simulink model "adsorption1"  (R2022b)
settings: Solver=VariableStepAuto  StartTime=0.0  StopTime=3600  RelTol=1e-3
libraries: fl_lib x171, nesl_utility x44
(part 1 of 2)
settings Model: Creator=kulka  LastModifiedBy=kulka

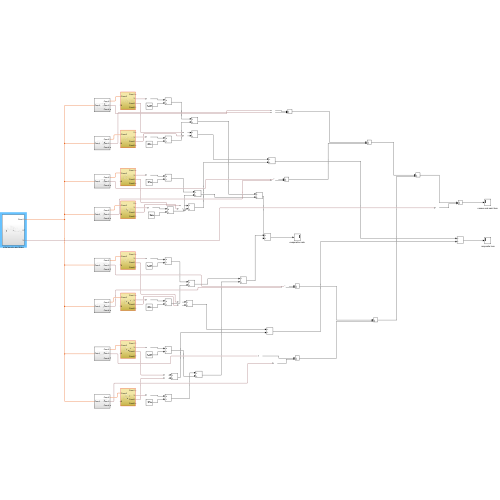
[thumbnail: Simulink's stored preview of the top-level diagram]
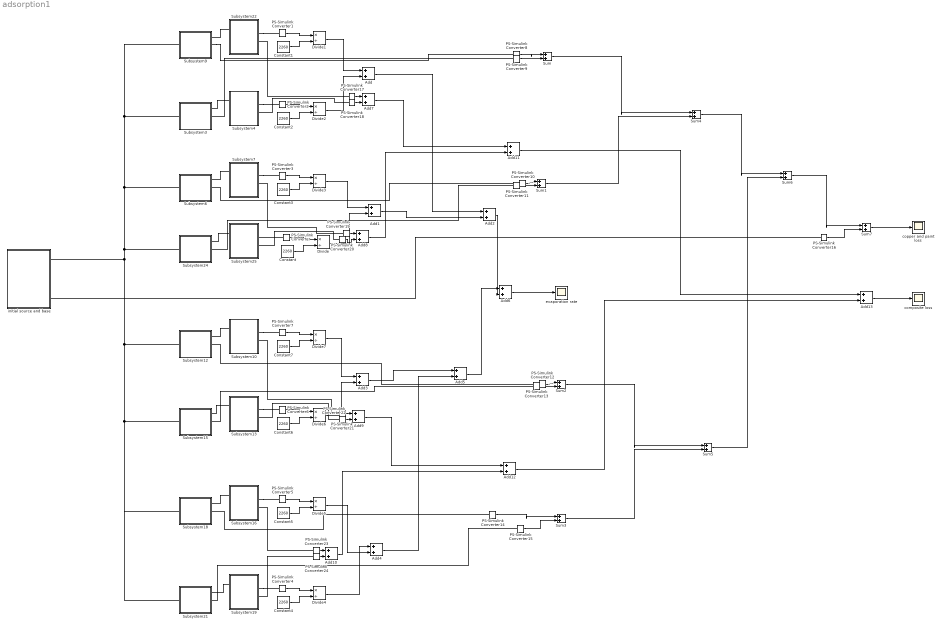
== system adsorption1 ==
  Add{,1..13} (14 alike) : Sum
  Constant{,1..7} (8 alike) : Constant  Value=2260
  Divide{,1..7} (8 alike) : Product  Inputs=*/  RndMeth=Zero  SaturateOnIntegerOverflow=on
  PS-Simulink Converter{,1..24} (25 alike) : nesl_utility/PS-Simulink Converter  PhysicalDomain=network_engine_domain  SubClassName=ps_output  LeftPortType=input  RightPortType=output  PseudoPeriodic=off  Frequencies=[]  VectorFormat=inherit  Unit=inherit  AffineConversion=off
  Subsystem10 : Subsystem
  Subsystem12 : Subsystem
  Subsystem13 : Subsystem
  Subsystem15 : Subsystem
  Subsystem16 : Subsystem
  Subsystem18 : Subsystem
  Subsystem19 : Subsystem
  Subsystem21 : Subsystem
  Subsystem22 : Subsystem
  Subsystem24 : Subsystem
  Subsystem25 : Subsystem
  Subsystem3 : Subsystem
  Subsystem4 : Subsystem
  Subsystem6 : Subsystem
  Subsystem7 : Subsystem
  Subsystem9 : Subsystem
  Sum{,1..7} (8 alike) : Sum  Inputs=|++
  composite loss : Scope
  copper and paint loss : Scope
  evaporation rate : Scope
  initial source and base : Subsystem
  wires:
  Constant/1 -> Divide/2
  PS-Simulink Converter/1 -> Divide/1
  PS-Simulink Converter1/1 -> Divide1/1
  Constant1/1 -> Divide1/2
  PS-Simulink Converter2/1 -> Divide2/1
  Constant2/1 -> Divide2/2
  PS-Simulink Converter3/1 -> Divide3/1
  Constant3/1 -> Divide3/2
  PS-Simulink Converter4/1 -> Divide4/1
  Constant4/1 -> Divide4/2
  PS-Simulink Converter5/1 -> Divide5/1
  Constant5/1 -> Divide5/2
  PS-Simulink Converter6/1 -> Divide6/1
  Constant6/1 -> Divide6/2
  PS-Simulink Converter7/1 -> Divide7/1
  Constant7/1 -> Divide7/2
  Divide1/1 -> Add/1
  Divide2/1 -> Add/2
  Divide3/1 -> Add1/1
  Divide/1 -> Add1/2
  Add/1 -> Add2/1
  Add1/1 -> Add2/2
  Divide7/1 -> Add3/1
  Divide6/1 -> Add3/2
  Divide5/1 -> Add4/2
  Divide4/1 -> Add4/1
  Add4/1 -> Add5/2
  Add3/1 -> Add5/1
  Add2/1 -> Add6/2
  Add5/1 -> Add6/1
  Add6/1 -> evaporation rate/1
  PS-Simulink Converter8/1 -> Sum/1
  PS-Simulink Converter9/1 -> Sum/2
  PS-Simulink Converter10/1 -> Sum1/1
  PS-Simulink Converter11/1 -> Sum1/2
  Sum/1 -> Sum4/1
  Sum1/1 -> Sum4/2
  Sum4/1 -> Sum6/1
  PS-Simulink Converter12/1 -> Sum2/1
  PS-Simulink Converter13/1 -> Sum2/2
  PS-Simulink Converter14/1 -> Sum3/1
  PS-Simulink Converter15/1 -> Sum3/2
  Sum3/1 -> Sum5/2
  Sum2/1 -> Sum5/1
  Sum5/1 -> Sum6/2
  Sum6/1 -> Sum7/1
  PS-Simulink Converter16/1 -> Sum7/2
  Sum7/1 -> copper and paint loss/1
  Add13/1 -> composite loss/1
  PS-Simulink Converter17/1 -> Add7/1
  PS-Simulink Converter18/1 -> Add7/2
  Add7/1 -> Add11/1
  PS-Simulink Converter19/1 -> Add8/1
  PS-Simulink Converter20/1 -> Add8/2
  Add8/1 -> Add11/2
  Add11/1 -> Add13/1
  PS-Simulink Converter21/1 -> Add9/1
  PS-Simulink Converter22/1 -> Add9/2
  Add9/1 -> Add12/1
  PS-Simulink Converter23/1 -> Add10/1
  PS-Simulink Converter24/1 -> Add10/2
  Add10/1 -> Add12/2
  Add12/1 -> Add13/2
  connections:
  Subsystem22/LConn1 -- Subsystem9/RConn1
  Subsystem4/LConn1 -- Subsystem3/RConn1
  Subsystem7/LConn1 -- Subsystem6/RConn1
  Subsystem25/LConn1 -- Subsystem24/RConn1
  Subsystem10/LConn1 -- Subsystem12/RConn1
  Subsystem13/LConn1 -- Subsystem15/RConn1
  Subsystem16/LConn1 -- Subsystem18/RConn1
  Subsystem21/LConn1 -- Subsystem18/LConn1 -- Subsystem15/LConn1 -- Subsystem12/LConn1 -- Subsystem24/LConn1 -- Subsystem6/LConn1 -- Subsystem9/LConn1 -- Subsystem3/LConn1 -- initial source and base/RConn1
  Subsystem19/LConn1 -- Subsystem21/RConn1
  PS-Simulink Converter/LConn1 -- Subsystem25/RConn2
  Subsystem22/RConn2 -- PS-Simulink Converter1/LConn1
  Subsystem4/RConn2 -- PS-Simulink Converter2/LConn1
  Subsystem7/RConn2 -- PS-Simulink Converter3/LConn1
  Subsystem19/RConn2 -- PS-Simulink Converter4/LConn1
  Subsystem16/RConn2 -- PS-Simulink Converter5/LConn1
  Subsystem13/RConn2 -- PS-Simulink Converter6/LConn1
  Subsystem10/RConn2 -- PS-Simulink Converter7/LConn1
  Subsystem9/RConn2 -- PS-Simulink Converter8/LConn1
  PS-Simulink Converter9/LConn1 -- Subsystem3/RConn2
  PS-Simulink Converter10/LConn1 -- Subsystem6/RConn2
  PS-Simulink Converter11/LConn1 -- Subsystem24/RConn2
  PS-Simulink Converter12/LConn1 -- Subsystem12/RConn2
  PS-Simulink Converter13/LConn1 -- Subsystem15/RConn2
  PS-Simulink Converter14/LConn1 -- Subsystem18/RConn2
  PS-Simulink Converter15/LConn1 -- Subsystem21/RConn2
  PS-Simulink Converter16/LConn1 -- initial source and base/RConn3
  PS-Simulink Converter17/LConn1 -- Subsystem22/RConn3
  PS-Simulink Converter18/LConn1 -- Subsystem4/RConn3
  PS-Simulink Converter19/LConn1 -- Subsystem7/RConn3
  PS-Simulink Converter20/LConn1 -- Subsystem25/RConn3
  PS-Simulink Converter21/LConn1 -- Subsystem10/RConn3
  PS-Simulink Converter22/LConn1 -- Subsystem13/RConn3
  PS-Simulink Converter23/LConn1 -- Subsystem16/RConn3
  PS-Simulink Converter24/LConn1 -- Subsystem19/RConn3

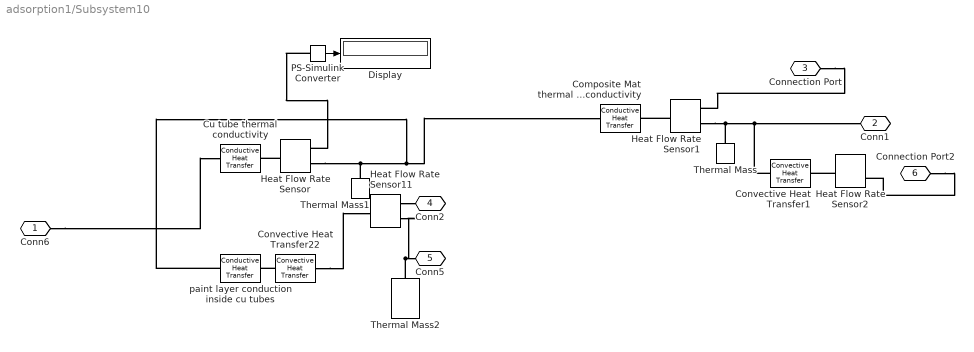
== system adsorption1/Subsystem10 ==
  Composite Mat thermal conductivity : fl_lib/Thermal/Thermal Elements/Conductive Heat Transfer  thermal_type=foundation.enum.ConstantVariableTabulated.Constant  wall_geometry=foundation.enum.ConductionWallGeometry.Planar  area=4186.1715e-6 m^2  thickness=0.002 m  d_in=0.05 m  d_out=0.1 m  L=1 m  th_cond_min=10 W/(K*m)  th_cond=0.1 W/(K*m)  th_cond_TLU=[413, 401, 392, 383, 371, 357, 342] W/(K*m)  temp_TLU=[200, 273, 400, 600, 800, 1000, 1200] K  T_specify=off  T_priority=None  T=0 K  T_nominal_specify=off  T_nominal_unit=K  T_nominal_value=1  Q_specify=on  Q_priority=None  Q=0 W  Q_nominal_specify=on  Q_nominal_unit=W  Q_nominal_value=1
  Convective Heat Transfer1 : fl_lib/Thermal/Thermal Elements/Convective Heat Transfer  thermal_type=foundation.enum.constant_variable.constant  area=4186.1715e-6 m^2  heat_tr_coeff=8 W/(K*m^2)  min_heat_tr_coeff=1e-3 W/(K*m^2)  T_specify=off  T_priority=None  T=0 K  T_nominal_specify=off  T_nominal_unit=K  T_nominal_value=1  Q_specify=on  Q_priority=None  Q=0 W  Q_nominal_specify=on  Q_nominal_unit=W  Q_nominal_value=1
  Convective Heat Transfer22 : fl_lib/Thermal/Thermal Elements/Convective Heat Transfer  thermal_type=foundation.enum.constant_variable.constant  area=3086.6125e-6 m^2  heat_tr_coeff=20 W/(K*m^2)  min_heat_tr_coeff=1e-3 W/(K*m^2)  T_specify=off  T_priority=None  T=0 K  T_nominal_specify=off  T_nominal_unit=K  T_nominal_value=1  Q_specify=on  Q_priority=None  Q=0 W  Q_nominal_specify=on  Q_nominal_unit=W  Q_nominal_value=1
  Cu tube thermal conductivity : fl_lib/Thermal/Thermal Elements/Conductive Heat Transfer  thermal_type=foundation.enum.ConstantVariableTabulated.Constant  wall_geometry=foundation.enum.ConductionWallGeometry.Planar  area=1.3744e-4 m^2  thickness=0.07 m  d_in=0.05 m  d_out=0.1 m  L=1 m  th_cond_min=10 W/(K*m)  th_cond=398 W/(K*m)  th_cond_TLU=[413, 401, 392, 383, 371, 357, 342] W/(K*m)  temp_TLU=[200, 273, 400, 600, 800, 1000, 1200] K  T_specify=off  T_priority=None  T=0 K  T_nominal_specify=off  T_nominal_unit=K  T_nominal_value=1  Q_specify=on  Q_priority=None  Q=0 W  Q_nominal_specify=on  Q_nominal_unit=W  Q_nominal_value=1
  Display : Display
  Heat Flow Rate Sensor{,1..2,11} (4 alike) : fl_lib/Thermal/Thermal Sensors/Heat Flow Rate Sensor
  PS-Simulink Converter : nesl_utility/PS-Simulink Converter  PhysicalDomain=network_engine_domain  SubClassName=ps_output  LeftPortType=input  RightPortType=output  PseudoPeriodic=off  Frequencies=[]  VectorFormat=inherit  Unit=inherit  AffineConversion=off
  Thermal Mass : fl_lib/Thermal/Thermal Elements/Thermal Mass  mass=6.6727e-2 kg  sp_heat=150 J/(K*kg)  num_ports=foundation.enum.numPorts2.one  T_specify=off  T_priority=High  T=300 K  T_nominal_specify=off  T_nominal_unit=K  T_nominal_value=1  Q_specify=off  Q_priority=None  Q=0 W  Q_nominal_specify=off  Q_nominal_unit=W  Q_nominal_value=1
  Thermal Mass1 : fl_lib/Thermal/Thermal Elements/Thermal Mass  mass=3.7865e-2 kg  sp_heat=390 J/(K*kg)  num_ports=foundation.enum.numPorts2.one  T_specify=off  T_priority=High  T=300 K  T_nominal_specify=off  T_nominal_unit=K  T_nominal_value=1  Q_specify=off  Q_priority=None  Q=0 W  Q_nominal_specify=off  Q_nominal_unit=W  Q_nominal_value=1
  Thermal Mass2 : fl_lib/Thermal/Thermal Elements/Thermal Mass  mass=0.001 kg  sp_heat=1000 J/(K*kg)  num_ports=foundation.enum.numPorts2.one  T_specify=off  T_priority=High  T=300 K  T_nominal_specify=off  T_nominal_unit=K  T_nominal_value=1  Q_specify=off  Q_priority=None  Q=0 W  Q_nominal_specify=off  Q_nominal_unit=W  Q_nominal_value=1
  paint layer conduction inside cu tubes : fl_lib/Thermal/Thermal Elements/Conductive Heat Transfer  thermal_type=foundation.enum.ConstantVariableTabulated.Constant  wall_geometry=foundation.enum.ConductionWallGeometry.Planar  area=3086.6125e-5 m^2  thickness=0.001 m  d_in=0.05 m  d_out=0.1 m  L=1 m  th_cond_min=10 W/(K*m)  th_cond=0.1 W/(K*m)  th_cond_TLU=[413, 401, 392, 383, 371, 357, 342] W/(K*m)  temp_TLU=[200, 273, 400, 600, 800, 1000, 1200] K  T_specify=off  T_priority=None  T=0 K  T_nominal_specify=off  T_nominal_unit=K  T_nominal_value=1  Q_specify=on  Q_priority=None  Q=0 W  Q_nominal_specify=on  Q_nominal_unit=W  Q_nominal_value=1
  Conn6 : PMIOPort  Side=Left
  Conn1 : PMIOPort  Port=2  Side=Right
  Connection Port : PMIOPort  Port=3  Side=Right
  Conn2 : PMIOPort  Port=4  Side=Right
  Conn5 : PMIOPort  Port=5  Side=Right
  Connection Port2 : PMIOPort  Port=6  Side=Left
  wires:
  PS-Simulink Converter/1 -> Display/1
  connections:
  Heat Flow Rate Sensor11/RConn1 -- Conn2/RConn1
  Conn6/RConn1 -- Cu tube thermal conductivity/LConn1
  Heat Flow Rate Sensor11/RConn2 -- Thermal Mass2/LConn1 -- Conn5/RConn1
  Convective Heat Transfer22/RConn1 -- Heat Flow Rate Sensor11/LConn1
  Convective Heat Transfer22/LConn1 -- paint layer conduction inside cu tubes/RConn1
  Heat Flow Rate Sensor/LConn1 -- Cu tube thermal conductivity/RConn1
  PS-Simulink Converter/LConn1 -- Heat Flow Rate Sensor/RConn1
  Heat Flow Rate Sensor/RConn2 -- Thermal Mass1/LConn1 -- paint layer conduction inside cu tubes/LConn1 -- Composite Mat thermal conductivity/LConn1
  Heat Flow Rate Sensor1/LConn1 -- Composite Mat thermal conductivity/RConn1
  Heat Flow Rate Sensor1/RConn2 -- Thermal Mass/LConn1 -- Convective Heat Transfer1/LConn1 -- Conn1/RConn1
  Connection Port/RConn1 -- Heat Flow Rate Sensor1/RConn1
  Connection Port2/RConn1 -- Heat Flow Rate Sensor2/RConn2
  Heat Flow Rate Sensor2/LConn1 -- Convective Heat Transfer1/RConn1

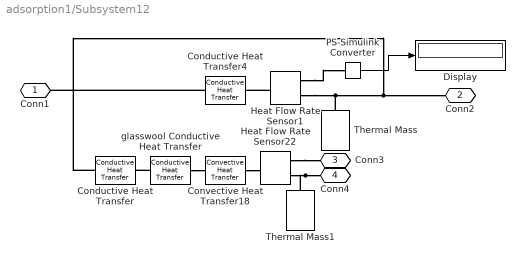
== system adsorption1/Subsystem12 ==
  Conductive Heat Transfer : fl_lib/Thermal/Thermal Elements/Conductive Heat Transfer  thermal_type=foundation.enum.ConstantVariableTabulated.Constant  wall_geometry=foundation.enum.ConductionWallGeometry.Planar  area=1.14e-3 m^2  thickness=0.02 m  d_in=0.05 m  d_out=0.1 m  L=1 m  th_cond_min=10 W/(K*m)  th_cond=0.1 W/(K*m)  th_cond_TLU=[413, 401, 392, 383, 371, 357, 342] W/(K*m)  temp_TLU=[200, 273, 400, 600, 800, 1000, 1200] K  T_specify=off  T_priority=None  T=0 K  T_nominal_specify=off  T_nominal_unit=K  T_nominal_value=1  Q_specify=on  Q_priority=None  Q=0 W  Q_nominal_specify=on  Q_nominal_unit=W  Q_nominal_value=1
  Conductive Heat Transfer4 : fl_lib/Thermal/Thermal Elements/Conductive Heat Transfer  thermal_type=foundation.enum.ConstantVariableTabulated.Constant  wall_geometry=foundation.enum.ConductionWallGeometry.Planar  area=1.14e-3 m^2  thickness=0.02 m  d_in=0.05 m  d_out=0.1 m  L=1 m  th_cond_min=10 W/(K*m)  th_cond=398 W/(K*m)  th_cond_TLU=[413, 401, 392, 383, 371, 357, 342] W/(K*m)  temp_TLU=[200, 273, 400, 600, 800, 1000, 1200] K  T_specify=off  T_priority=None  T=0 K  T_nominal_specify=off  T_nominal_unit=K  T_nominal_value=1  Q_specify=on  Q_priority=None  Q=0 W  Q_nominal_specify=on  Q_nominal_unit=W  Q_nominal_value=1
  Convective Heat Transfer18 : fl_lib/Thermal/Thermal Elements/Convective Heat Transfer  thermal_type=foundation.enum.constant_variable.constant  area=1.14e-3 m^2  heat_tr_coeff=12 W/(K*m^2)  min_heat_tr_coeff=1e-3 W/(K*m^2)  T_specify=off  T_priority=None  T=0 K  T_nominal_specify=off  T_nominal_unit=K  T_nominal_value=1  Q_specify=on  Q_priority=None  Q=0 W  Q_nominal_specify=on  Q_nominal_unit=W  Q_nominal_value=1
  Display : Display
  Heat Flow Rate Sensor1 : fl_lib/Thermal/Thermal Sensors/Heat Flow Rate Sensor
  Heat Flow Rate Sensor22 : fl_lib/Thermal/Thermal Sensors/Heat Flow Rate Sensor
  PS-Simulink Converter : nesl_utility/PS-Simulink Converter  PhysicalDomain=network_engine_domain  SubClassName=ps_output  LeftPortType=input  RightPortType=output  PseudoPeriodic=off  Frequencies=[]  VectorFormat=inherit  Unit=inherit  AffineConversion=off
  Thermal Mass : fl_lib/Thermal/Thermal Elements/Thermal Mass  mass=(0.20178)-(1.885e-6) kg  sp_heat=390 J/(K*kg)  num_ports=foundation.enum.numPorts2.one  T_specify=off  T_priority=High  T=300 K  T_nominal_specify=off  T_nominal_unit=K  T_nominal_value=1  Q_specify=off  Q_priority=None  Q=0 W  Q_nominal_specify=off  Q_nominal_unit=W  Q_nominal_value=1
  Thermal Mass1 : fl_lib/Thermal/Thermal Elements/Thermal Mass  mass=0.001 kg  sp_heat=1000 J/(K*kg)  num_ports=foundation.enum.numPorts2.one  T_specify=off  T_priority=High  T=300 K  T_nominal_specify=off  T_nominal_unit=K  T_nominal_value=1  Q_specify=off  Q_priority=None  Q=0 W  Q_nominal_specify=off  Q_nominal_unit=W  Q_nominal_value=1
  glasswool Conductive Heat Transfer : fl_lib/Thermal/Thermal Elements/Conductive Heat Transfer  thermal_type=foundation.enum.ConstantVariableTabulated.Constant  wall_geometry=foundation.enum.ConductionWallGeometry.Planar  area=3e-3 m^2  thickness=5e-3 m  d_in=0.05 m  d_out=0.1 m  L=1 m  th_cond_min=10 W/(K*m)  th_cond=0.032 W/(K*m)  th_cond_TLU=[413, 401, 392, 383, 371, 357, 342] W/(K*m)  temp_TLU=[200, 273, 400, 600, 800, 1000, 1200] K  T_specify=off  T_priority=None  T=0 K  T_nominal_specify=off  T_nominal_unit=K  T_nominal_value=1  Q_specify=on  Q_priority=None  Q=0 W  Q_nominal_specify=on  Q_nominal_unit=W  Q_nominal_value=1
  Conn1 : PMIOPort  Side=Left
  Conn2 : PMIOPort  Port=2  Side=Right
  Conn3 : PMIOPort  Port=3  Side=Right
  Conn4 : PMIOPort  Port=4  Side=Right
  wires:
  PS-Simulink Converter/1 -> Display/1
  connections:
  Conductive Heat Transfer4/LConn1 -- Conn1/RConn1
  Convective Heat Transfer18/RConn1 -- Heat Flow Rate Sensor22/LConn1
  Heat Flow Rate Sensor22/RConn2 -- Thermal Mass1/LConn1 -- Conn4/RConn1
  Heat Flow Rate Sensor22/RConn1 -- Conn3/RConn1
  Heat Flow Rate Sensor1/LConn1 -- Conductive Heat Transfer4/RConn1
  Heat Flow Rate Sensor1/RConn2 -- Thermal Mass/LConn1 -- Conductive Heat Transfer/LConn1 -- Conn2/RConn1
  Heat Flow Rate Sensor1/RConn1 -- PS-Simulink Converter/LConn1
  glasswool Conductive Heat Transfer/LConn1 -- Conductive Heat Transfer/RConn1
  glasswool Conductive Heat Transfer/RConn1 -- Convective Heat Transfer18/LConn1

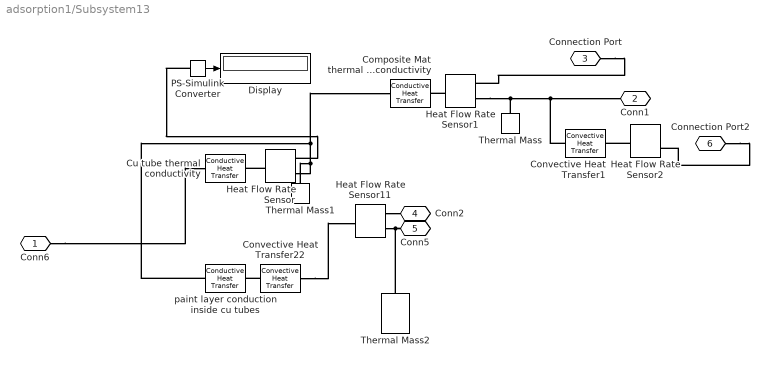
== system adsorption1/Subsystem13 ==
  Composite Mat thermal conductivity : fl_lib/Thermal/Thermal Elements/Conductive Heat Transfer  thermal_type=foundation.enum.ConstantVariableTabulated.Constant  wall_geometry=foundation.enum.ConductionWallGeometry.Planar  area=4186.1715e-6 m^2  thickness=0.002 m  d_in=0.05 m  d_out=0.1 m  L=1 m  th_cond_min=10 W/(K*m)  th_cond=0.1 W/(K*m)  th_cond_TLU=[413, 401, 392, 383, 371, 357, 342] W/(K*m)  temp_TLU=[200, 273, 400, 600, 800, 1000, 1200] K  T_specify=off  T_priority=None  T=0 K  T_nominal_specify=off  T_nominal_unit=K  T_nominal_value=1  Q_specify=on  Q_priority=None  Q=0 W  Q_nominal_specify=on  Q_nominal_unit=W  Q_nominal_value=1
  Convective Heat Transfer1 : fl_lib/Thermal/Thermal Elements/Convective Heat Transfer  thermal_type=foundation.enum.constant_variable.constant  area=4186.1715e-6 m^2  heat_tr_coeff=8 W/(K*m^2)  min_heat_tr_coeff=1e-3 W/(K*m^2)  T_specify=off  T_priority=None  T=0 K  T_nominal_specify=off  T_nominal_unit=K  T_nominal_value=1  Q_specify=on  Q_priority=None  Q=0 W  Q_nominal_specify=on  Q_nominal_unit=W  Q_nominal_value=1
  Convective Heat Transfer22 : fl_lib/Thermal/Thermal Elements/Convective Heat Transfer  thermal_type=foundation.enum.constant_variable.constant  area=3086.6125e-6 m^2  heat_tr_coeff=20 W/(K*m^2)  min_heat_tr_coeff=1e-3 W/(K*m^2)  T_specify=off  T_priority=None  T=0 K  T_nominal_specify=off  T_nominal_unit=K  T_nominal_value=1  Q_specify=on  Q_priority=None  Q=0 W  Q_nominal_specify=on  Q_nominal_unit=W  Q_nominal_value=1
  Cu tube thermal conductivity : fl_lib/Thermal/Thermal Elements/Conductive Heat Transfer  thermal_type=foundation.enum.ConstantVariableTabulated.Constant  wall_geometry=foundation.enum.ConductionWallGeometry.Planar  area=1.3744e-4 m^2  thickness=0.07 m  d_in=0.05 m  d_out=0.1 m  L=1 m  th_cond_min=10 W/(K*m)  th_cond=398 W/(K*m)  th_cond_TLU=[413, 401, 392, 383, 371, 357, 342] W/(K*m)  temp_TLU=[200, 273, 400, 600, 800, 1000, 1200] K  T_specify=off  T_priority=None  T=0 K  T_nominal_specify=off  T_nominal_unit=K  T_nominal_value=1  Q_specify=on  Q_priority=None  Q=0 W  Q_nominal_specify=on  Q_nominal_unit=W  Q_nominal_value=1
  Display : Display
  Heat Flow Rate Sensor{,1..2,11} (4 alike) : fl_lib/Thermal/Thermal Sensors/Heat Flow Rate Sensor
  PS-Simulink Converter : nesl_utility/PS-Simulink Converter  PhysicalDomain=network_engine_domain  SubClassName=ps_output  LeftPortType=input  RightPortType=output  PseudoPeriodic=off  Frequencies=[]  VectorFormat=inherit  Unit=inherit  AffineConversion=off
  Thermal Mass : fl_lib/Thermal/Thermal Elements/Thermal Mass  mass=6.6727e-2 kg  sp_heat=150 J/(K*kg)  num_ports=foundation.enum.numPorts2.one  T_specify=off  T_priority=High  T=300 K  T_nominal_specify=off  T_nominal_unit=K  T_nominal_value=1  Q_specify=off  Q_priority=None  Q=0 W  Q_nominal_specify=off  Q_nominal_unit=W  Q_nominal_value=1
  Thermal Mass1 : fl_lib/Thermal/Thermal Elements/Thermal Mass  mass=3.7865e-2 kg  sp_heat=390 J/(K*kg)  num_ports=foundation.enum.numPorts2.one  T_specify=off  T_priority=High  T=300 K  T_nominal_specify=off  T_nominal_unit=K  T_nominal_value=1  Q_specify=off  Q_priority=None  Q=0 W  Q_nominal_specify=off  Q_nominal_unit=W  Q_nominal_value=1
  Thermal Mass2 : fl_lib/Thermal/Thermal Elements/Thermal Mass  mass=0.001 kg  sp_heat=1000 J/(K*kg)  num_ports=foundation.enum.numPorts2.one  T_specify=off  T_priority=High  T=300 K  T_nominal_specify=off  T_nominal_unit=K  T_nominal_value=1  Q_specify=off  Q_priority=None  Q=0 W  Q_nominal_specify=off  Q_nominal_unit=W  Q_nominal_value=1
  paint layer conduction inside cu tubes : fl_lib/Thermal/Thermal Elements/Conductive Heat Transfer  thermal_type=foundation.enum.ConstantVariableTabulated.Constant  wall_geometry=foundation.enum.ConductionWallGeometry.Planar  area=3086.6125e-5 m^2  thickness=0.001 m  d_in=0.05 m  d_out=0.1 m  L=1 m  th_cond_min=10 W/(K*m)  th_cond=0.1 W/(K*m)  th_cond_TLU=[413, 401, 392, 383, 371, 357, 342] W/(K*m)  temp_TLU=[200, 273, 400, 600, 800, 1000, 1200] K  T_specify=off  T_priority=None  T=0 K  T_nominal_specify=off  T_nominal_unit=K  T_nominal_value=1  Q_specify=on  Q_priority=None  Q=0 W  Q_nominal_specify=on  Q_nominal_unit=W  Q_nominal_value=1
  Conn6 : PMIOPort  Side=Left
  Conn1 : PMIOPort  Port=2  Side=Right
  Connection Port : PMIOPort  Port=3  Side=Right
  Conn2 : PMIOPort  Port=4  Side=Right
  Conn5 : PMIOPort  Port=5  Side=Right
  Connection Port2 : PMIOPort  Port=6  Side=Left
  wires:
  PS-Simulink Converter/1 -> Display/1
  connections:
  Heat Flow Rate Sensor11/RConn1 -- Conn2/RConn1
  Conn6/RConn1 -- Cu tube thermal conductivity/LConn1
  Heat Flow Rate Sensor11/RConn2 -- Thermal Mass2/LConn1 -- Conn5/RConn1
  Convective Heat Transfer22/RConn1 -- Heat Flow Rate Sensor11/LConn1
  Convective Heat Transfer22/LConn1 -- paint layer conduction inside cu tubes/RConn1
  Heat Flow Rate Sensor/LConn1 -- Cu tube thermal conductivity/RConn1
  PS-Simulink Converter/LConn1 -- Heat Flow Rate Sensor/RConn1
  Heat Flow Rate Sensor/RConn2 -- Thermal Mass1/LConn1 -- paint layer conduction inside cu tubes/LConn1 -- Composite Mat thermal conductivity/LConn1
  Heat Flow Rate Sensor1/LConn1 -- Composite Mat thermal conductivity/RConn1
  Heat Flow Rate Sensor1/RConn2 -- Thermal Mass/LConn1 -- Convective Heat Transfer1/LConn1 -- Conn1/RConn1
  Connection Port/RConn1 -- Heat Flow Rate Sensor1/RConn1
  Connection Port2/RConn1 -- Heat Flow Rate Sensor2/RConn2
  Heat Flow Rate Sensor2/LConn1 -- Convective Heat Transfer1/RConn1

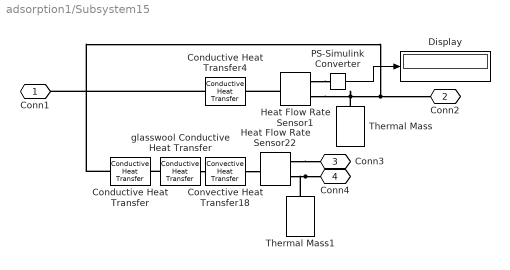
== system adsorption1/Subsystem15 ==
  Conductive Heat Transfer : fl_lib/Thermal/Thermal Elements/Conductive Heat Transfer  thermal_type=foundation.enum.ConstantVariableTabulated.Constant  wall_geometry=foundation.enum.ConductionWallGeometry.Planar  area=2*1.14e-3 m^2  thickness=0.02*2 m  d_in=0.05 m  d_out=0.1 m  L=1 m  th_cond_min=10 W/(K*m)  th_cond=0.1 W/(K*m)  th_cond_TLU=[413, 401, 392, 383, 371, 357, 342] W/(K*m)  temp_TLU=[200, 273, 400, 600, 800, 1000, 1200] K  T_specify=off  T_priority=None  T=0 K  T_nominal_specify=off  T_nominal_unit=K  T_nominal_value=1  Q_specify=on  Q_priority=None  Q=0 W  Q_nominal_specify=on  Q_nominal_unit=W  Q_nominal_value=1
  Conductive Heat Transfer4 : fl_lib/Thermal/Thermal Elements/Conductive Heat Transfer  thermal_type=foundation.enum.ConstantVariableTabulated.Constant  wall_geometry=foundation.enum.ConductionWallGeometry.Planar  area=2*1.14e-3 m^2  thickness=0.02*2 m  d_in=0.05 m  d_out=0.1 m  L=1 m  th_cond_min=10 W/(K*m)  th_cond=398 W/(K*m)  th_cond_TLU=[413, 401, 392, 383, 371, 357, 342] W/(K*m)  temp_TLU=[200, 273, 400, 600, 800, 1000, 1200] K  T_specify=off  T_priority=None  T=0 K  T_nominal_specify=off  T_nominal_unit=K  T_nominal_value=1  Q_specify=on  Q_priority=None  Q=0 W  Q_nominal_specify=on  Q_nominal_unit=W  Q_nominal_value=1
  Convective Heat Transfer18 : fl_lib/Thermal/Thermal Elements/Convective Heat Transfer  thermal_type=foundation.enum.constant_variable.constant  area=1.14e-3 m^2  heat_tr_coeff=12 W/(K*m^2)  min_heat_tr_coeff=1e-3 W/(K*m^2)  T_specify=off  T_priority=None  T=0 K  T_nominal_specify=off  T_nominal_unit=K  T_nominal_value=1  Q_specify=on  Q_priority=None  Q=0 W  Q_nominal_specify=on  Q_nominal_unit=W  Q_nominal_value=1
  Display : Display
  Heat Flow Rate Sensor1 : fl_lib/Thermal/Thermal Sensors/Heat Flow Rate Sensor
  Heat Flow Rate Sensor22 : fl_lib/Thermal/Thermal Sensors/Heat Flow Rate Sensor
  PS-Simulink Converter : nesl_utility/PS-Simulink Converter  PhysicalDomain=network_engine_domain  SubClassName=ps_output  LeftPortType=input  RightPortType=output  PseudoPeriodic=off  Frequencies=[]  VectorFormat=inherit  Unit=inherit  AffineConversion=off
  Thermal Mass : fl_lib/Thermal/Thermal Elements/Thermal Mass  mass=(2*0.20178)-(2*1.885e-6) kg  sp_heat=390 J/(K*kg)  num_ports=foundation.enum.numPorts2.one  T_specify=off  T_priority=High  T=300 K  T_nominal_specify=off  T_nominal_unit=K  T_nominal_value=1  Q_specify=off  Q_priority=None  Q=0 W  Q_nominal_specify=off  Q_nominal_unit=W  Q_nominal_value=1
  Thermal Mass1 : fl_lib/Thermal/Thermal Elements/Thermal Mass  mass=0.001 kg  sp_heat=1000 J/(K*kg)  num_ports=foundation.enum.numPorts2.one  T_specify=off  T_priority=High  T=300 K  T_nominal_specify=off  T_nominal_unit=K  T_nominal_value=1  Q_specify=off  Q_priority=None  Q=0 W  Q_nominal_specify=off  Q_nominal_unit=W  Q_nominal_value=1
  glasswool Conductive Heat Transfer : fl_lib/Thermal/Thermal Elements/Conductive Heat Transfer  thermal_type=foundation.enum.ConstantVariableTabulated.Constant  wall_geometry=foundation.enum.ConductionWallGeometry.Planar  area=3e-3 m^2  thickness=5e-3 m  d_in=0.05 m  d_out=0.1 m  L=1 m  th_cond_min=10 W/(K*m)  th_cond=0.032 W/(K*m)  th_cond_TLU=[413, 401, 392, 383, 371, 357, 342] W/(K*m)  temp_TLU=[200, 273, 400, 600, 800, 1000, 1200] K  T_specify=off  T_priority=None  T=0 K  T_nominal_specify=off  T_nominal_unit=K  T_nominal_value=1  Q_specify=on  Q_priority=None  Q=0 W  Q_nominal_specify=on  Q_nominal_unit=W  Q_nominal_value=1
  Conn1 : PMIOPort  Side=Left
  Conn2 : PMIOPort  Port=2  Side=Right
  Conn3 : PMIOPort  Port=3  Side=Right
  Conn4 : PMIOPort  Port=4  Side=Right
  wires:
  PS-Simulink Converter/1 -> Display/1
  connections:
  Conductive Heat Transfer4/LConn1 -- Conn1/RConn1
  Convective Heat Transfer18/RConn1 -- Heat Flow Rate Sensor22/LConn1
  Heat Flow Rate Sensor22/RConn2 -- Thermal Mass1/LConn1 -- Conn4/RConn1
  Heat Flow Rate Sensor22/RConn1 -- Conn3/RConn1
  Heat Flow Rate Sensor1/LConn1 -- Conductive Heat Transfer4/RConn1
  Heat Flow Rate Sensor1/RConn2 -- Thermal Mass/LConn1 -- Conductive Heat Transfer/LConn1 -- Conn2/RConn1
  Heat Flow Rate Sensor1/RConn1 -- PS-Simulink Converter/LConn1
  glasswool Conductive Heat Transfer/LConn1 -- Conductive Heat Transfer/RConn1
  glasswool Conductive Heat Transfer/RConn1 -- Convective Heat Transfer18/LConn1

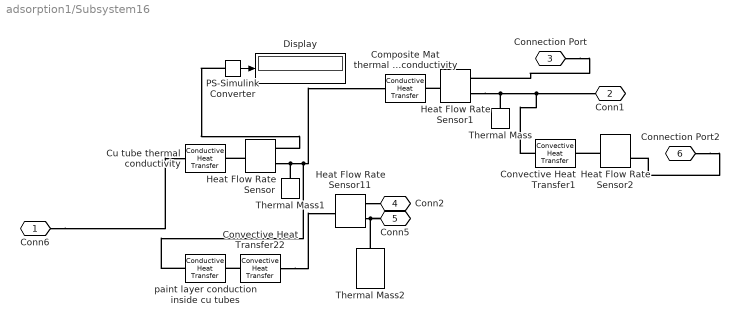
== system adsorption1/Subsystem16 ==
  Composite Mat thermal conductivity : fl_lib/Thermal/Thermal Elements/Conductive Heat Transfer  thermal_type=foundation.enum.ConstantVariableTabulated.Constant  wall_geometry=foundation.enum.ConductionWallGeometry.Planar  area=4186.1715e-6 m^2  thickness=0.002 m  d_in=0.05 m  d_out=0.1 m  L=1 m  th_cond_min=10 W/(K*m)  th_cond=0.1 W/(K*m)  th_cond_TLU=[413, 401, 392, 383, 371, 357, 342] W/(K*m)  temp_TLU=[200, 273, 400, 600, 800, 1000, 1200] K  T_specify=off  T_priority=None  T=0 K  T_nominal_specify=off  T_nominal_unit=K  T_nominal_value=1  Q_specify=on  Q_priority=None  Q=0 W  Q_nominal_specify=on  Q_nominal_unit=W  Q_nominal_value=1
  Convective Heat Transfer1 : fl_lib/Thermal/Thermal Elements/Convective Heat Transfer  thermal_type=foundation.enum.constant_variable.constant  area=4186.1715e-6 m^2  heat_tr_coeff=8 W/(K*m^2)  min_heat_tr_coeff=1e-3 W/(K*m^2)  T_specify=off  T_priority=None  T=0 K  T_nominal_specify=off  T_nominal_unit=K  T_nominal_value=1  Q_specify=on  Q_priority=None  Q=0 W  Q_nominal_specify=on  Q_nominal_unit=W  Q_nominal_value=1
  Convective Heat Transfer22 : fl_lib/Thermal/Thermal Elements/Convective Heat Transfer  thermal_type=foundation.enum.constant_variable.constant  area=3086.6125e-6 m^2  heat_tr_coeff=20 W/(K*m^2)  min_heat_tr_coeff=1e-3 W/(K*m^2)  T_specify=off  T_priority=None  T=0 K  T_nominal_specify=off  T_nominal_unit=K  T_nominal_value=1  Q_specify=on  Q_priority=None  Q=0 W  Q_nominal_specify=on  Q_nominal_unit=W  Q_nominal_value=1
  Cu tube thermal conductivity : fl_lib/Thermal/Thermal Elements/Conductive Heat Transfer  thermal_type=foundation.enum.ConstantVariableTabulated.Constant  wall_geometry=foundation.enum.ConductionWallGeometry.Planar  area=1.3744e-4 m^2  thickness=0.07 m  d_in=0.05 m  d_out=0.1 m  L=1 m  th_cond_min=10 W/(K*m)  th_cond=398 W/(K*m)  th_cond_TLU=[413, 401, 392, 383, 371, 357, 342] W/(K*m)  temp_TLU=[200, 273, 400, 600, 800, 1000, 1200] K  T_specify=off  T_priority=None  T=0 K  T_nominal_specify=off  T_nominal_unit=K  T_nominal_value=1  Q_specify=on  Q_priority=None  Q=0 W  Q_nominal_specify=on  Q_nominal_unit=W  Q_nominal_value=1
  Display : Display
  Heat Flow Rate Sensor{,1..2,11} (4 alike) : fl_lib/Thermal/Thermal Sensors/Heat Flow Rate Sensor
  PS-Simulink Converter : nesl_utility/PS-Simulink Converter  PhysicalDomain=network_engine_domain  SubClassName=ps_output  LeftPortType=input  RightPortType=output  PseudoPeriodic=off  Frequencies=[]  VectorFormat=inherit  Unit=inherit  AffineConversion=off
  Thermal Mass : fl_lib/Thermal/Thermal Elements/Thermal Mass  mass=6.6727e-2 kg  sp_heat=150 J/(K*kg)  num_ports=foundation.enum.numPorts2.one  T_specify=off  T_priority=High  T=300 K  T_nominal_specify=off  T_nominal_unit=K  T_nominal_value=1  Q_specify=off  Q_priority=None  Q=0 W  Q_nominal_specify=off  Q_nominal_unit=W  Q_nominal_value=1
  Thermal Mass1 : fl_lib/Thermal/Thermal Elements/Thermal Mass  mass=3.7865e-2 kg  sp_heat=390 J/(K*kg)  num_ports=foundation.enum.numPorts2.one  T_specify=off  T_priority=High  T=300 K  T_nominal_specify=off  T_nominal_unit=K  T_nominal_value=1  Q_specify=off  Q_priority=None  Q=0 W  Q_nominal_specify=off  Q_nominal_unit=W  Q_nominal_value=1
  Thermal Mass2 : fl_lib/Thermal/Thermal Elements/Thermal Mass  mass=0.001 kg  sp_heat=1000 J/(K*kg)  num_ports=foundation.enum.numPorts2.one  T_specify=off  T_priority=High  T=300 K  T_nominal_specify=off  T_nominal_unit=K  T_nominal_value=1  Q_specify=off  Q_priority=None  Q=0 W  Q_nominal_specify=off  Q_nominal_unit=W  Q_nominal_value=1
  paint layer conduction inside cu tubes : fl_lib/Thermal/Thermal Elements/Conductive Heat Transfer  thermal_type=foundation.enum.ConstantVariableTabulated.Constant  wall_geometry=foundation.enum.ConductionWallGeometry.Planar  area=3086.6125e-5 m^2  thickness=0.001 m  d_in=0.05 m  d_out=0.1 m  L=1 m  th_cond_min=10 W/(K*m)  th_cond=0.1 W/(K*m)  th_cond_TLU=[413, 401, 392, 383, 371, 357, 342] W/(K*m)  temp_TLU=[200, 273, 400, 600, 800, 1000, 1200] K  T_specify=off  T_priority=None  T=0 K  T_nominal_specify=off  T_nominal_unit=K  T_nominal_value=1  Q_specify=on  Q_priority=None  Q=0 W  Q_nominal_specify=on  Q_nominal_unit=W  Q_nominal_value=1
  Conn6 : PMIOPort  Side=Left
  Conn1 : PMIOPort  Port=2  Side=Right
  Connection Port : PMIOPort  Port=3  Side=Right
  Conn2 : PMIOPort  Port=4  Side=Right
  Conn5 : PMIOPort  Port=5  Side=Right
  Connection Port2 : PMIOPort  Port=6  Side=Left
  wires:
  PS-Simulink Converter/1 -> Display/1
  connections:
  Heat Flow Rate Sensor11/RConn1 -- Conn2/RConn1
  Conn6/RConn1 -- Cu tube thermal conductivity/LConn1
  Heat Flow Rate Sensor11/RConn2 -- Thermal Mass2/LConn1 -- Conn5/RConn1
  Convective Heat Transfer22/RConn1 -- Heat Flow Rate Sensor11/LConn1
  Convective Heat Transfer22/LConn1 -- paint layer conduction inside cu tubes/RConn1
  Heat Flow Rate Sensor/LConn1 -- Cu tube thermal conductivity/RConn1
  PS-Simulink Converter/LConn1 -- Heat Flow Rate Sensor/RConn1
  Heat Flow Rate Sensor/RConn2 -- Thermal Mass1/LConn1 -- paint layer conduction inside cu tubes/LConn1 -- Composite Mat thermal conductivity/LConn1
  Heat Flow Rate Sensor1/LConn1 -- Composite Mat thermal conductivity/RConn1
  Heat Flow Rate Sensor1/RConn2 -- Thermal Mass/LConn1 -- Convective Heat Transfer1/LConn1 -- Conn1/RConn1
  Connection Port/RConn1 -- Heat Flow Rate Sensor1/RConn1
  Connection Port2/RConn1 -- Heat Flow Rate Sensor2/RConn2
  Heat Flow Rate Sensor2/LConn1 -- Convective Heat Transfer1/RConn1

== system adsorption1/Subsystem18 ==
  Conductive Heat Transfer : fl_lib/Thermal/Thermal Elements/Conductive Heat Transfer  thermal_type=foundation.enum.ConstantVariableTabulated.Constant  wall_geometry=foundation.enum.ConductionWallGeometry.Planar  area=3*1.14e-3 m^2  thickness=0.02*3 m  d_in=0.05 m  d_out=0.1 m  L=1 m  th_cond_min=10 W/(K*m)  th_cond=0.1 W/(K*m)  th_cond_TLU=[413, 401, 392, 383, 371, 357, 342] W/(K*m)  temp_TLU=[200, 273, 400, 600, 800, 1000, 1200] K  T_specify=off  T_priority=None  T=0 K  T_nominal_specify=off  T_nominal_unit=K  T_nominal_value=1  Q_specify=on  Q_priority=None  Q=0 W  Q_nominal_specify=on  Q_nominal_unit=W  Q_nominal_value=1
  Conductive Heat Transfer4 : fl_lib/Thermal/Thermal Elements/Conductive Heat Transfer  thermal_type=foundation.enum.ConstantVariableTabulated.Constant  wall_geometry=foundation.enum.ConductionWallGeometry.Planar  area=3*1.14e-3 m^2  thickness=0.02*3 m  d_in=0.05 m  d_out=0.1 m  L=1 m  th_cond_min=10 W/(K*m)  th_cond=398 W/(K*m)  th_cond_TLU=[413, 401, 392, 383, 371, 357, 342] W/(K*m)  temp_TLU=[200, 273, 400, 600, 800, 1000, 1200] K  T_specify=off  T_priority=None  T=0 K  T_nominal_specify=off  T_nominal_unit=K  T_nominal_value=1  Q_specify=on  Q_priority=None  Q=0 W  Q_nominal_specify=on  Q_nominal_unit=W  Q_nominal_value=1
  Convective Heat Transfer18 : fl_lib/Thermal/Thermal Elements/Convective Heat Transfer  thermal_type=foundation.enum.constant_variable.constant  area=1.14e-3 m^2  heat_tr_coeff=12 W/(K*m^2)  min_heat_tr_coeff=1e-3 W/(K*m^2)  T_specify=off  T_priority=None  T=0 K  T_nominal_specify=off  T_nominal_unit=K  T_nominal_value=1  Q_specify=on  Q_priority=None  Q=0 W  Q_nominal_specify=on  Q_nominal_unit=W  Q_nominal_value=1
  Display : Display
  Heat Flow Rate Sensor1 : fl_lib/Thermal/Thermal Sensors/Heat Flow Rate Sensor
  Heat Flow Rate Sensor22 : fl_lib/Thermal/Thermal Sensors/Heat Flow Rate Sensor
  PS-Simulink Converter : nesl_utility/PS-Simulink Converter  PhysicalDomain=network_engine_domain  SubClassName=ps_output  LeftPortType=input  RightPortType=output  PseudoPeriodic=off  Frequencies=[]  VectorFormat=inherit  Unit=inherit  AffineConversion=off
  Thermal Mass : fl_lib/Thermal/Thermal Elements/Thermal Mass  mass=(3*0.20178)-(3*1.885e-6) kg  sp_heat=390 J/(K*kg)  num_ports=foundation.enum.numPorts2.one  T_specify=off  T_priority=High  T=300 K  T_nominal_specify=off  T_nominal_unit=K  T_nominal_value=1  Q_specify=off  Q_priority=None  Q=0 W  Q_nominal_specify=off  Q_nominal_unit=W  Q_nominal_value=1
  Thermal Mass1 : fl_lib/Thermal/Thermal Elements/Thermal Mass  mass=0.001 kg  sp_heat=1000 J/(K*kg)  num_ports=foundation.enum.numPorts2.one  T_specify=off  T_priority=High  T=300 K  T_nominal_specify=off  T_nominal_unit=K  T_nominal_value=1  Q_specify=off  Q_priority=None  Q=0 W  Q_nominal_specify=off  Q_nominal_unit=W  Q_nominal_value=1
  glasswool Conductive Heat Transfer : fl_lib/Thermal/Thermal Elements/Conductive Heat Transfer  thermal_type=foundation.enum.ConstantVariableTabulated.Constant  wall_geometry=foundation.enum.ConductionWallGeometry.Planar  area=3e-3 m^2  thickness=5e-3 m  d_in=0.05 m  d_out=0.1 m  L=1 m  th_cond_min=10 W/(K*m)  th_cond=0.032 W/(K*m)  th_cond_TLU=[413, 401, 392, 383, 371, 357, 342] W/(K*m)  temp_TLU=[200, 273, 400, 600, 800, 1000, 1200] K  T_specify=off  T_priority=None  T=0 K  T_nominal_specify=off  T_nominal_unit=K  T_nominal_value=1  Q_specify=on  Q_priority=None  Q=0 W  Q_nominal_specify=on  Q_nominal_unit=W  Q_nominal_value=1
  Conn1 : PMIOPort  Side=Left
  Conn2 : PMIOPort  Port=2  Side=Right
  Conn3 : PMIOPort  Port=3  Side=Right
  Conn4 : PMIOPort  Port=4  Side=Right
  wires:
  PS-Simulink Converter/1 -> Display/1
  connections:
  Conductive Heat Transfer4/LConn1 -- Conn1/RConn1
  Convective Heat Transfer18/RConn1 -- Heat Flow Rate Sensor22/LConn1
  Heat Flow Rate Sensor22/RConn2 -- Thermal Mass1/LConn1 -- Conn4/RConn1
  Heat Flow Rate Sensor22/RConn1 -- Conn3/RConn1
  Heat Flow Rate Sensor1/LConn1 -- Conductive Heat Transfer4/RConn1
  Heat Flow Rate Sensor1/RConn2 -- Thermal Mass/LConn1 -- Conductive Heat Transfer/LConn1 -- Conn2/RConn1
  Heat Flow Rate Sensor1/RConn1 -- PS-Simulink Converter/LConn1
  glasswool Conductive Heat Transfer/LConn1 -- Conductive Heat Transfer/RConn1
  glasswool Conductive Heat Transfer/RConn1 -- Convective Heat Transfer18/LConn1

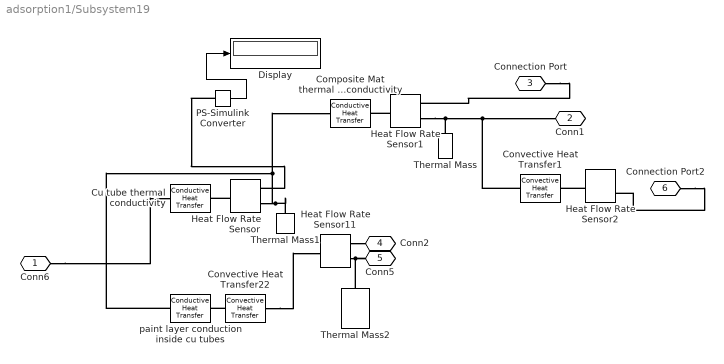
== system adsorption1/Subsystem19 ==
  Composite Mat thermal conductivity : fl_lib/Thermal/Thermal Elements/Conductive Heat Transfer  thermal_type=foundation.enum.ConstantVariableTabulated.Constant  wall_geometry=foundation.enum.ConductionWallGeometry.Planar  area=4186.1715e-6 m^2  thickness=0.002 m  d_in=0.05 m  d_out=0.1 m  L=1 m  th_cond_min=10 W/(K*m)  th_cond=0.1 W/(K*m)  th_cond_TLU=[413, 401, 392, 383, 371, 357, 342] W/(K*m)  temp_TLU=[200, 273, 400, 600, 800, 1000, 1200] K  T_specify=off  T_priority=None  T=0 K  T_nominal_specify=off  T_nominal_unit=K  T_nominal_value=1  Q_specify=on  Q_priority=None  Q=0 W  Q_nominal_specify=on  Q_nominal_unit=W  Q_nominal_value=1
  Convective Heat Transfer1 : fl_lib/Thermal/Thermal Elements/Convective Heat Transfer  thermal_type=foundation.enum.constant_variable.constant  area=4186.1715e-6 m^2  heat_tr_coeff=8 W/(K*m^2)  min_heat_tr_coeff=1e-3 W/(K*m^2)  T_specify=off  T_priority=None  T=0 K  T_nominal_specify=off  T_nominal_unit=K  T_nominal_value=1  Q_specify=on  Q_priority=None  Q=0 W  Q_nominal_specify=on  Q_nominal_unit=W  Q_nominal_value=1
  Convective Heat Transfer22 : fl_lib/Thermal/Thermal Elements/Convective Heat Transfer  thermal_type=foundation.enum.constant_variable.constant  area=3086.6125e-6 m^2  heat_tr_coeff=20 W/(K*m^2)  min_heat_tr_coeff=1e-3 W/(K*m^2)  T_specify=off  T_priority=None  T=0 K  T_nominal_specify=off  T_nominal_unit=K  T_nominal_value=1  Q_specify=on  Q_priority=None  Q=0 W  Q_nominal_specify=on  Q_nominal_unit=W  Q_nominal_value=1
  Cu tube thermal conductivity : fl_lib/Thermal/Thermal Elements/Conductive Heat Transfer  thermal_type=foundation.enum.ConstantVariableTabulated.Constant  wall_geometry=foundation.enum.ConductionWallGeometry.Planar  area=1.3744e-4 m^2  thickness=0.07 m  d_in=0.05 m  d_out=0.1 m  L=1 m  th_cond_min=10 W/(K*m)  th_cond=398 W/(K*m)  th_cond_TLU=[413, 401, 392, 383, 371, 357, 342] W/(K*m)  temp_TLU=[200, 273, 400, 600, 800, 1000, 1200] K  T_specify=off  T_priority=None  T=0 K  T_nominal_specify=off  T_nominal_unit=K  T_nominal_value=1  Q_specify=on  Q_priority=None  Q=0 W  Q_nominal_specify=on  Q_nominal_unit=W  Q_nominal_value=1
  Display : Display
  Heat Flow Rate Sensor{,1..2,11} (4 alike) : fl_lib/Thermal/Thermal Sensors/Heat Flow Rate Sensor
  PS-Simulink Converter : nesl_utility/PS-Simulink Converter  PhysicalDomain=network_engine_domain  SubClassName=ps_output  LeftPortType=input  RightPortType=output  PseudoPeriodic=off  Frequencies=[]  VectorFormat=inherit  Unit=inherit  AffineConversion=off
  Thermal Mass : fl_lib/Thermal/Thermal Elements/Thermal Mass  mass=6.6727e-2 kg  sp_heat=150 J/(K*kg)  num_ports=foundation.enum.numPorts2.one  T_specify=off  T_priority=High  T=300 K  T_nominal_specify=off  T_nominal_unit=K  T_nominal_value=1  Q_specify=off  Q_priority=None  Q=0 W  Q_nominal_specify=off  Q_nominal_unit=W  Q_nominal_value=1
  Thermal Mass1 : fl_lib/Thermal/Thermal Elements/Thermal Mass  mass=3.7865e-2 kg  sp_heat=390 J/(K*kg)  num_ports=foundation.enum.numPorts2.one  T_specify=off  T_priority=High  T=300 K  T_nominal_specify=off  T_nominal_unit=K  T_nominal_value=1  Q_specify=off  Q_priority=None  Q=0 W  Q_nominal_specify=off  Q_nominal_unit=W  Q_nominal_value=1
  Thermal Mass2 : fl_lib/Thermal/Thermal Elements/Thermal Mass  mass=0.001 kg  sp_heat=1000 J/(K*kg)  num_ports=foundation.enum.numPorts2.one  T_specify=off  T_priority=High  T=300 K  T_nominal_specify=off  T_nominal_unit=K  T_nominal_value=1  Q_specify=off  Q_priority=None  Q=0 W  Q_nominal_specify=off  Q_nominal_unit=W  Q_nominal_value=1
  paint layer conduction inside cu tubes : fl_lib/Thermal/Thermal Elements/Conductive Heat Transfer  thermal_type=foundation.enum.ConstantVariableTabulated.Constant  wall_geometry=foundation.enum.ConductionWallGeometry.Planar  area=3086.6125e-5 m^2  thickness=0.001 m  d_in=0.05 m  d_out=0.1 m  L=1 m  th_cond_min=10 W/(K*m)  th_cond=0.1 W/(K*m)  th_cond_TLU=[413, 401, 392, 383, 371, 357, 342] W/(K*m)  temp_TLU=[200, 273, 400, 600, 800, 1000, 1200] K  T_specify=off  T_priority=None  T=0 K  T_nominal_specify=off  T_nominal_unit=K  T_nominal_value=1  Q_specify=on  Q_priority=None  Q=0 W  Q_nominal_specify=on  Q_nominal_unit=W  Q_nominal_value=1
  Conn6 : PMIOPort  Side=Left
  Conn1 : PMIOPort  Port=2  Side=Right
  Connection Port : PMIOPort  Port=3  Side=Right
  Conn2 : PMIOPort  Port=4  Side=Right
  Conn5 : PMIOPort  Port=5  Side=Right
  Connection Port2 : PMIOPort  Port=6  Side=Left
  wires:
  PS-Simulink Converter/1 -> Display/1
  connections:
  Heat Flow Rate Sensor11/RConn1 -- Conn2/RConn1
  Conn6/RConn1 -- Cu tube thermal conductivity/LConn1
  Heat Flow Rate Sensor11/RConn2 -- Thermal Mass2/LConn1 -- Conn5/RConn1
  Convective Heat Transfer22/RConn1 -- Heat Flow Rate Sensor11/LConn1
  Convective Heat Transfer22/LConn1 -- paint layer conduction inside cu tubes/RConn1
  Heat Flow Rate Sensor/LConn1 -- Cu tube thermal conductivity/RConn1
  PS-Simulink Converter/LConn1 -- Heat Flow Rate Sensor/RConn1
  Heat Flow Rate Sensor/RConn2 -- paint layer conduction inside cu tubes/LConn1 -- Composite Mat thermal conductivity/LConn1 -- Thermal Mass1/LConn1
  Heat Flow Rate Sensor1/LConn1 -- Composite Mat thermal conductivity/RConn1
  Heat Flow Rate Sensor1/RConn2 -- Thermal Mass/LConn1 -- Convective Heat Transfer1/LConn1 -- Conn1/RConn1
  Connection Port/RConn1 -- Heat Flow Rate Sensor1/RConn1
  Connection Port2/RConn1 -- Heat Flow Rate Sensor2/RConn2
  Heat Flow Rate Sensor2/LConn1 -- Convective Heat Transfer1/RConn1

== system adsorption1/Subsystem21 ==
  Conductive Heat Transfer : fl_lib/Thermal/Thermal Elements/Conductive Heat Transfer  thermal_type=foundation.enum.ConstantVariableTabulated.Constant  wall_geometry=foundation.enum.ConductionWallGeometry.Planar  area=4*1.14e-3 m^2  thickness=0.02*4 + 0.01 m  d_in=0.05 m  d_out=0.1 m  L=1 m  th_cond_min=10 W/(K*m)  th_cond=0.1 W/(K*m)  th_cond_TLU=[413, 401, 392, 383, 371, 357, 342] W/(K*m)  temp_TLU=[200, 273, 400, 600, 800, 1000, 1200] K  T_specify=off  T_priority=None  T=0 K  T_nominal_specify=off  T_nominal_unit=K  T_nominal_value=1  Q_specify=on  Q_priority=None  Q=0 W  Q_nominal_specify=on  Q_nominal_unit=W  Q_nominal_value=1
  Conductive Heat Transfer4 : fl_lib/Thermal/Thermal Elements/Conductive Heat Transfer  thermal_type=foundation.enum.ConstantVariableTabulated.Constant  wall_geometry=foundation.enum.ConductionWallGeometry.Planar  area=4*1.14e-3 m^2  thickness=0.02*4 + 0.01 m  d_in=0.05 m  d_out=0.1 m  L=1 m  th_cond_min=10 W/(K*m)  th_cond=398 W/(K*m)  th_cond_TLU=[413, 401, 392, 383, 371, 357, 342] W/(K*m)  temp_TLU=[200, 273, 400, 600, 800, 1000, 1200] K  T_specify=off  T_priority=None  T=0 K  T_nominal_specify=off  T_nominal_unit=K  T_nominal_value=1  Q_specify=on  Q_priority=None  Q=0 W  Q_nominal_specify=on  Q_nominal_unit=W  Q_nominal_value=1
  Convective Heat Transfer18 : fl_lib/Thermal/Thermal Elements/Convective Heat Transfer  thermal_type=foundation.enum.constant_variable.constant  area=1.14e-3 m^2  heat_tr_coeff=12 W/(K*m^2)  min_heat_tr_coeff=1e-3 W/(K*m^2)  T_specify=off  T_priority=None  T=0 K  T_nominal_specify=off  T_nominal_unit=K  T_nominal_value=1  Q_specify=on  Q_priority=None  Q=0 W  Q_nominal_specify=on  Q_nominal_unit=W  Q_nominal_value=1
  Display : Display
  Heat Flow Rate Sensor1 : fl_lib/Thermal/Thermal Sensors/Heat Flow Rate Sensor
  Heat Flow Rate Sensor22 : fl_lib/Thermal/Thermal Sensors/Heat Flow Rate Sensor
  PS-Simulink Converter : nesl_utility/PS-Simulink Converter  PhysicalDomain=network_engine_domain  SubClassName=ps_output  LeftPortType=input  RightPortType=output  PseudoPeriodic=off  Frequencies=[]  VectorFormat=inherit  Unit=inherit  AffineConversion=off
  Thermal Mass : fl_lib/Thermal/Thermal Elements/Thermal Mass  mass=(4*0.20178)-(4*1.885e-6) kg  sp_heat=390 J/(K*kg)  num_ports=foundation.enum.numPorts2.one  T_specify=off  T_priority=High  T=300 K  T_nominal_specify=off  T_nominal_unit=K  T_nominal_value=1  Q_specify=off  Q_priority=None  Q=0 W  Q_nominal_specify=off  Q_nominal_unit=W  Q_nominal_value=1
  Thermal Mass1 : fl_lib/Thermal/Thermal Elements/Thermal Mass  mass=0.001 kg  sp_heat=1000 J/(K*kg)  num_ports=foundation.enum.numPorts2.one  T_specify=off  T_priority=High  T=300 K  T_nominal_specify=off  T_nominal_unit=K  T_nominal_value=1  Q_specify=off  Q_priority=None  Q=0 W  Q_nominal_specify=off  Q_nominal_unit=W  Q_nominal_value=1
  glasswool Conductive Heat Transfer : fl_lib/Thermal/Thermal Elements/Conductive Heat Transfer  thermal_type=foundation.enum.ConstantVariableTabulated.Constant  wall_geometry=foundation.enum.ConductionWallGeometry.Planar  area=3e-3 m^2  thickness=5e-3 m  d_in=0.05 m  d_out=0.1 m  L=1 m  th_cond_min=10 W/(K*m)  th_cond=0.032 W/(K*m)  th_cond_TLU=[413, 401, 392, 383, 371, 357, 342] W/(K*m)  temp_TLU=[200, 273, 400, 600, 800, 1000, 1200] K  T_specify=off  T_priority=None  T=0 K  T_nominal_specify=off  T_nominal_unit=K  T_nominal_value=1  Q_specify=on  Q_priority=None  Q=0 W  Q_nominal_specify=on  Q_nominal_unit=W  Q_nominal_value=1
  Conn1 : PMIOPort  Side=Left
  Conn2 : PMIOPort  Port=2  Side=Right
  Conn3 : PMIOPort  Port=3  Side=Right
  Conn4 : PMIOPort  Port=4  Side=Right
  wires:
  PS-Simulink Converter/1 -> Display/1
  connections:
  Conductive Heat Transfer4/LConn1 -- Conn1/RConn1
  Convective Heat Transfer18/RConn1 -- Heat Flow Rate Sensor22/LConn1
  Heat Flow Rate Sensor22/RConn2 -- Thermal Mass1/LConn1 -- Conn4/RConn1
  Heat Flow Rate Sensor22/RConn1 -- Conn3/RConn1
  Heat Flow Rate Sensor1/LConn1 -- Conductive Heat Transfer4/RConn1
  Heat Flow Rate Sensor1/RConn2 -- Thermal Mass/LConn1 -- Conductive Heat Transfer/LConn1 -- Conn2/RConn1
  Heat Flow Rate Sensor1/RConn1 -- PS-Simulink Converter/LConn1
  glasswool Conductive Heat Transfer/LConn1 -- Conductive Heat Transfer/RConn1
  glasswool Conductive Heat Transfer/RConn1 -- Convective Heat Transfer18/LConn1
